simulink model "Neighborhood"  (R2024b)
settings: Solver=VariableStepAuto  StartTime=0.0  StopTime=20  RelTol=1e-3
undefined symbols (not defined in the file): A, A0_obv, adj, agent_1, agent_2, agent_3, agent_4, agent_5, agent_6, agent_noise_sensitivity_1, agent_noise_sensitivity_2, agent_noise_sensitivity_3, agent_noise_sensitivity_4, agent_noise_sensitivity_5, agent_noise_sensitivity_6, B, B0_obv, c, C, C0_obv, D, D0_obv, F, G, K, K0, noise_sensitivity, noise_ts
settings Model: Creator=Ivan  LastModifiedBy=Ivan

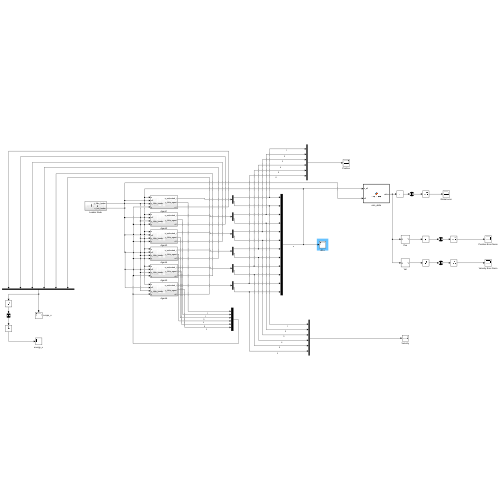
[thumbnail: Simulink's stored preview of the top-level diagram]
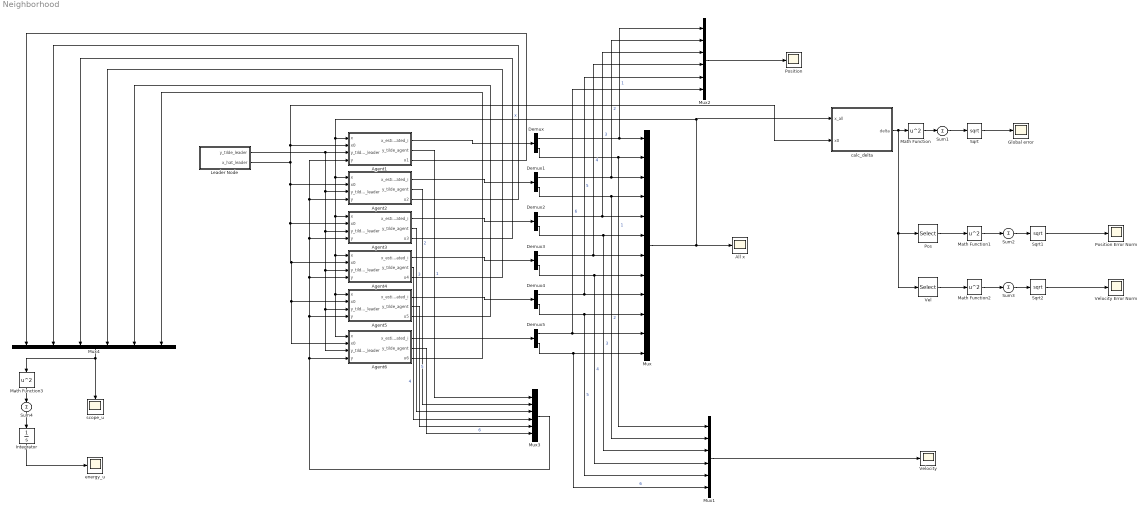
== system Neighborhood ==
  Agent1 : Subsystem
  Agent2 : Subsystem
  Agent3 : Subsystem
  Agent4 : Subsystem
  Agent5 : Subsystem
  Agent6 : Subsystem
  All x : Scope
  Demux{,1..5} (6 alike) : Demux  Outputs=2
  Global error : Scope
  Integrator : Integrator
  Leader Node : Subsystem
  Math Function{,1..3} (4 alike) : Math  Operator=square
  Mux : Mux  Inputs=12
  Mux{1..4} (4 alike) : Mux  Inputs=6
  Pos : Selector  NumberOfDimensions=2  InputPortWidth=3  IndexOptions=Index vector (dialog),Select all  Indices=[1],1  OutputSizes=1,1
  Position : Scope
  "Position Error Norm " : Scope
  Sqrt : Sqrt
  Sqrt1 : Sqrt
  Sqrt2 : Sqrt
  Sum{1..4} (4 alike) : Sum  Inputs=1
  Vel : Selector  NumberOfDimensions=2  InputPortWidth=3  IndexOptions=Index vector (dialog),Select all  Indices=[2],1  OutputSizes=1,1
  Velocity : Scope
  Velocity Error Norm : Scope
  calc_delta : MATLAB Function  TreatAsAtomicUnit=on
  energy_u : Scope
  scope_u : Scope
  wires:
  Demux1/2 -> Mux1/2, Mux/4  "2"
  Demux/1 -> Mux2/1, Mux/1  "1"
  Demux4/2 -> Mux1/5, Mux/10  "5"
  Demux/2 -> Mux/2, Mux1/1  "1"
  Demux1/1 -> Mux2/2, Mux/3  "2"
  Demux2/2 -> Mux1/3, Mux/6  "3"
  Demux4/1 -> Mux2/5, Mux/9  "5"
  Demux2/1 -> Mux/5, Mux2/3  "3"
  Demux3/2 -> Mux1/4, Mux/8  "4"
  Mux2/1 -> Position/1
  Mux1/1 -> Velocity/1
  Demux5/1 -> Mux2/6, Mux/11  "6"
  Demux5/2 -> Mux1/6, Mux/12  "6"
  Leader Node/2(x_hat_leader) -> calc_delta/2(x0), Agent1/2(x0), Agent2/2(x0), Agent3/2(x0), Agent4/2(x0), Agent6/2(x0), Agent5/2(x0)
  Mux/1 -> All x/1, calc_delta/1(x_all), Agent1/1(x), Agent2/1(x), Agent3/1(x), Agent4/1(x), Agent6/1(x), Agent5/1(x)  "x"
  Agent1/1(x_estimated_i) -> Demux/1
  Demux3/1 -> Mux2/4, Mux/7  "4"
  Agent2/1(x_estimated_i) -> Demux1/1
  Agent3/1(x_estimated_i) -> Demux2/1
  Agent4/1(x_estimated_i) -> Demux3/1
  Agent5/1(x_estimated_i) -> Demux4/1
  Agent6/1(x_estimated_i) -> Demux5/1
  Leader Node/1(y_tilde_leader) -> Agent2/3(y_tilde_leader), Agent3/3(y_tilde_leader), Agent4/3(y_tilde_leader), Agent6/3(y_tilde_leader), Agent5/3(y_tilde_leader), Agent1/3(y_tilde_leader)
  Agent1/2(y_tilde_agent) -> Mux3/1  "1"
  Agent2/2(y_tilde_agent) -> Mux3/2  "2"
  Agent3/2(y_tilde_agent) -> Mux3/3  "3"
  Agent4/2(y_tilde_agent) -> Mux3/4  "4"
  Agent5/2(y_tilde_agent) -> Mux3/5  "5"
  Agent6/2(y_tilde_agent) -> Mux3/6  "6"
  Mux3/1 -> Agent5/4(y), Agent4/4(y), Agent3/4(y), Agent2/4(y), Agent1/4(y), Agent6/4(y)
  Math Function2/1 -> Sum3/1
  Vel/1 -> Math Function2/1
  Sqrt/1 -> Global error/1
  Sum1/1 -> Sqrt/1
  Math Function1/1 -> Sum2/1
  Pos/1 -> Math Function1/1
  calc_delta/1(delta) -> Vel/1, Pos/1, Math Function/1
  Math Function/1 -> Sum1/1
  Sqrt2/1 -> Velocity Error Norm/1
  Sum3/1 -> Sqrt2/1
  Sum2/1 -> Sqrt1/1
  Sqrt1/1 -> "Position Error Norm "/1
  Sum4/1 -> Integrator/1
  Math Function3/1 -> Sum4/1
  Integrator/1 -> energy_u/1
  Mux4/1 -> scope_u/1, Math Function3/1
  Agent1/3(u1) -> Mux4/1
  Agent2/3(u2) -> Mux4/2
  Agent3/3(u3) -> Mux4/3
  Agent4/3(u4) -> Mux4/4
  Agent5/3(u5) -> Mux4/5
  Agent6/3(u6) -> Mux4/6

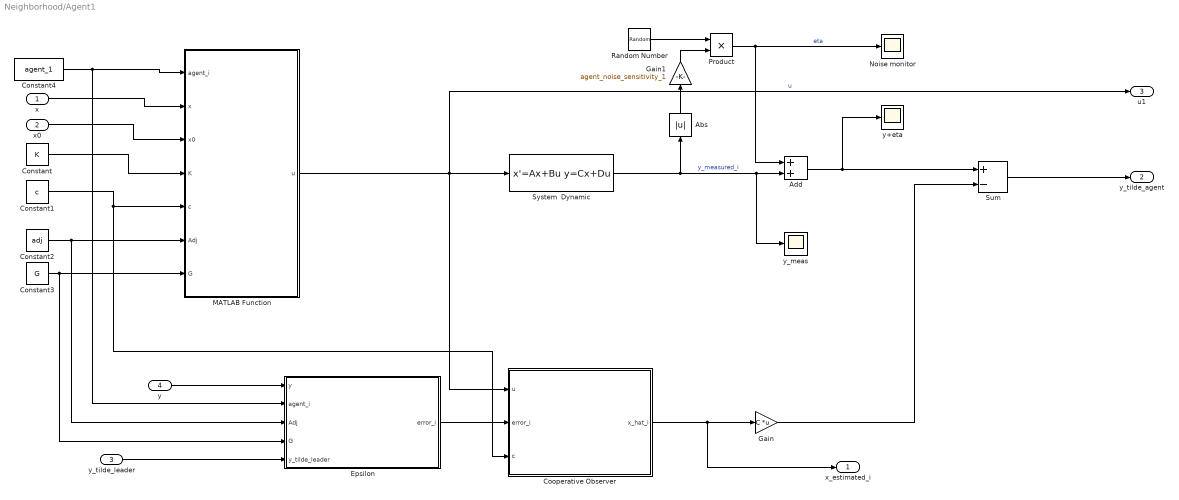
== system Neighborhood/Agent1 ==
  x : Inport
  x0 : Inport  Port=2
  y_tilde_leader : Inport  Port=3
  y : Inport  Port=4
  Abs : Abs  SaturateOnIntegerOverflow=off
  Add : Sum
  Constant : Constant  Value=K  VectorParams1D=off
  Constant1 : Constant  Value=c
  Constant2 : Constant  Value=adj
  Constant3 : Constant  Value=G
  Constant4 : Constant  Value=agent_1  VectorParams1D=off
  Cooperative Observer : Subsystem
  Epsilon : MATLAB Function  TreatAsAtomicUnit=on
  Gain : Gain  Gain=C  Multiplication=Matrix(K*u)
  Gain1 : Gain  Gain=agent_noise_sensitivity_1
  MATLAB Function : MATLAB Function  TreatAsAtomicUnit=on
  Noise monitor : Scope
  Product : Product
  Random Number : RandomNumber  SampleTime=noise_ts
  Sum : Sum  Inputs=+-
  System  Dynamic : StateSpace  A=(A-B*K0)  B=B  C=C  D=0  InitialCondition=0
  y+eta : Scope
  y_meas : Scope
  x_estimated_i : Outport
  y_tilde_agent : Outport  Port=2
  u1 : Outport  Port=3
  wires:
  x/1 -> MATLAB Function/2(x)
  Constant3/1 -> Epsilon/4(G), MATLAB Function/7(G)
  Constant1/1 -> Cooperative Observer/3(c), MATLAB Function/5(c)
  Constant/1 -> MATLAB Function/4(K)
  Constant4/1 -> Epsilon/2(agent_i), MATLAB Function/1(agent_i)
  Constant2/1 -> MATLAB Function/6(Adj), Epsilon/3(Adj)
  MATLAB Function/1(u) -> u1/1, Cooperative Observer/1(u), System  Dynamic/1  "u"
  x0/1 -> MATLAB Function/3(x0)
  y/1 -> Epsilon/1(y)
  y_tilde_leader/1 -> Epsilon/5(y_tilde_leader)
  Epsilon/1(error_i) -> Cooperative Observer/2(error_i)
  Cooperative Observer/1(x_hat_i) -> x_estimated_i/1, Gain/1
  System  Dynamic/1 -> Abs/1, y_meas/1, Add/2  "y_measured_i"
  Gain/1 -> Sum/2
  Sum/1 -> y_tilde_agent/1
  Product/1 -> Noise monitor/1, Add/1  "eta"
  Gain1/1 -> Product/2
  Abs/1 -> Gain1/1
  Random Number/1 -> Product/1
  Add/1 -> y+eta/1, Sum/1

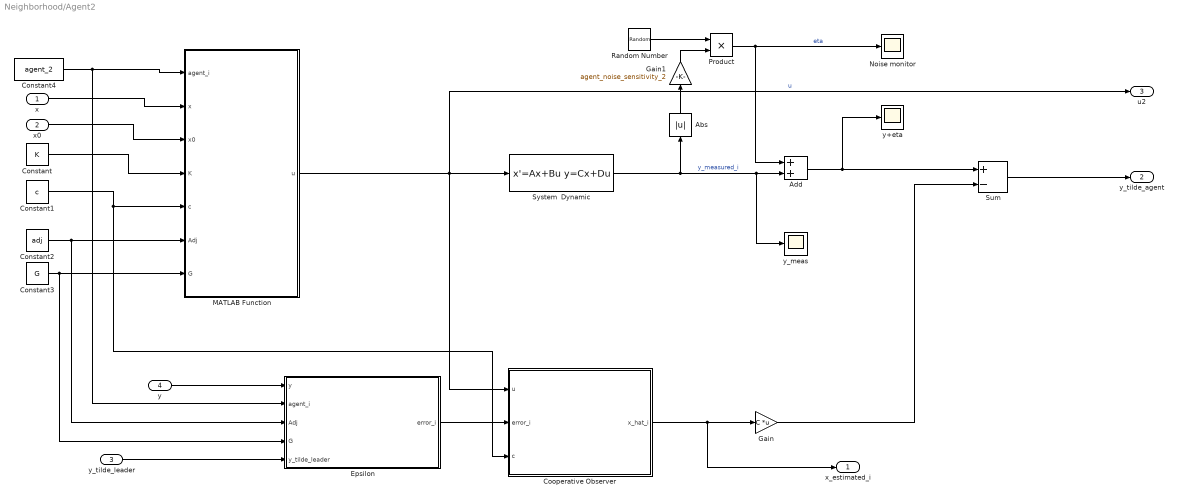
== system Neighborhood/Agent2 ==
  x : Inport
  x0 : Inport  Port=2
  y_tilde_leader : Inport  Port=3
  y : Inport  Port=4
  Abs : Abs  SaturateOnIntegerOverflow=off
  Add : Sum
  Constant : Constant  Value=K  VectorParams1D=off
  Constant1 : Constant  Value=c
  Constant2 : Constant  Value=adj
  Constant3 : Constant  Value=G
  Constant4 : Constant  Value=agent_2  VectorParams1D=off
  Cooperative Observer : Subsystem
  Epsilon : MATLAB Function  TreatAsAtomicUnit=on
  Gain : Gain  Gain=C  Multiplication=Matrix(K*u)
  Gain1 : Gain  Gain=agent_noise_sensitivity_2
  MATLAB Function : MATLAB Function  TreatAsAtomicUnit=on
  Noise monitor : Scope
  Product : Product
  Random Number : RandomNumber  SampleTime=noise_ts
  Sum : Sum  Inputs=+-
  System  Dynamic : StateSpace  A=(A-B*K0)  B=B  C=C  D=0  InitialCondition=0
  y+eta : Scope
  y_meas : Scope
  x_estimated_i : Outport
  y_tilde_agent : Outport  Port=2
  u2 : Outport  Port=3
  wires:
  x/1 -> MATLAB Function/2(x)
  Constant3/1 -> Epsilon/4(G), MATLAB Function/7(G)
  Constant1/1 -> Cooperative Observer/3(c), MATLAB Function/5(c)
  Constant/1 -> MATLAB Function/4(K)
  Constant4/1 -> Epsilon/2(agent_i), MATLAB Function/1(agent_i)
  Constant2/1 -> MATLAB Function/6(Adj), Epsilon/3(Adj)
  MATLAB Function/1(u) -> u2/1, Cooperative Observer/1(u), System  Dynamic/1  "u"
  x0/1 -> MATLAB Function/3(x0)
  y/1 -> Epsilon/1(y)
  y_tilde_leader/1 -> Epsilon/5(y_tilde_leader)
  Epsilon/1(error_i) -> Cooperative Observer/2(error_i)
  Cooperative Observer/1(x_hat_i) -> x_estimated_i/1, Gain/1
  System  Dynamic/1 -> Abs/1, y_meas/1, Add/2  "y_measured_i"
  Gain/1 -> Sum/2
  Sum/1 -> y_tilde_agent/1
  Product/1 -> Noise monitor/1, Add/1  "eta"
  Gain1/1 -> Product/2
  Abs/1 -> Gain1/1
  Random Number/1 -> Product/1
  Add/1 -> y+eta/1, Sum/1

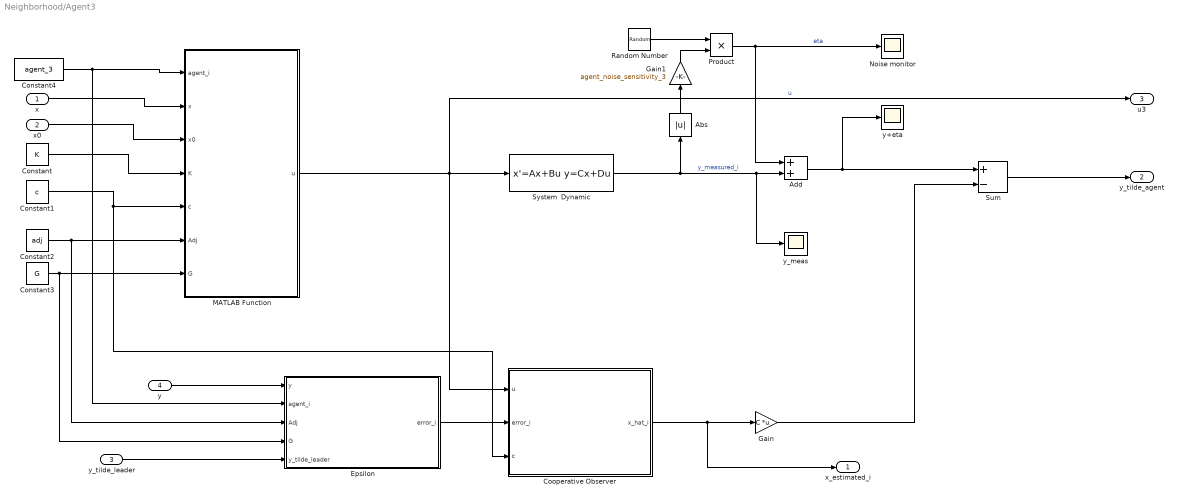
== system Neighborhood/Agent3 ==
  x : Inport
  x0 : Inport  Port=2
  y_tilde_leader : Inport  Port=3
  y : Inport  Port=4
  Abs : Abs  SaturateOnIntegerOverflow=off
  Add : Sum
  Constant : Constant  Value=K  VectorParams1D=off
  Constant1 : Constant  Value=c
  Constant2 : Constant  Value=adj
  Constant3 : Constant  Value=G
  Constant4 : Constant  Value=agent_3  VectorParams1D=off
  Cooperative Observer : Subsystem
  Epsilon : MATLAB Function  TreatAsAtomicUnit=on
  Gain : Gain  Gain=C  Multiplication=Matrix(K*u)
  Gain1 : Gain  Gain=agent_noise_sensitivity_3
  MATLAB Function : MATLAB Function  TreatAsAtomicUnit=on
  Noise monitor : Scope
  Product : Product
  Random Number : RandomNumber  SampleTime=noise_ts
  Sum : Sum  Inputs=+-
  System  Dynamic : StateSpace  A=(A-B*K0)  B=B  C=C  D=0  InitialCondition=0
  y+eta : Scope
  y_meas : Scope
  x_estimated_i : Outport
  y_tilde_agent : Outport  Port=2
  u3 : Outport  Port=3
  wires:
  x/1 -> MATLAB Function/2(x)
  Constant3/1 -> Epsilon/4(G), MATLAB Function/7(G)
  Constant1/1 -> Cooperative Observer/3(c), MATLAB Function/5(c)
  Constant/1 -> MATLAB Function/4(K)
  Constant4/1 -> Epsilon/2(agent_i), MATLAB Function/1(agent_i)
  Constant2/1 -> MATLAB Function/6(Adj), Epsilon/3(Adj)
  MATLAB Function/1(u) -> u3/1, Cooperative Observer/1(u), System  Dynamic/1  "u"
  x0/1 -> MATLAB Function/3(x0)
  y/1 -> Epsilon/1(y)
  y_tilde_leader/1 -> Epsilon/5(y_tilde_leader)
  Epsilon/1(error_i) -> Cooperative Observer/2(error_i)
  Cooperative Observer/1(x_hat_i) -> x_estimated_i/1, Gain/1
  System  Dynamic/1 -> Abs/1, y_meas/1, Add/2  "y_measured_i"
  Gain/1 -> Sum/2
  Sum/1 -> y_tilde_agent/1
  Product/1 -> Noise monitor/1, Add/1  "eta"
  Gain1/1 -> Product/2
  Abs/1 -> Gain1/1
  Random Number/1 -> Product/1
  Add/1 -> y+eta/1, Sum/1

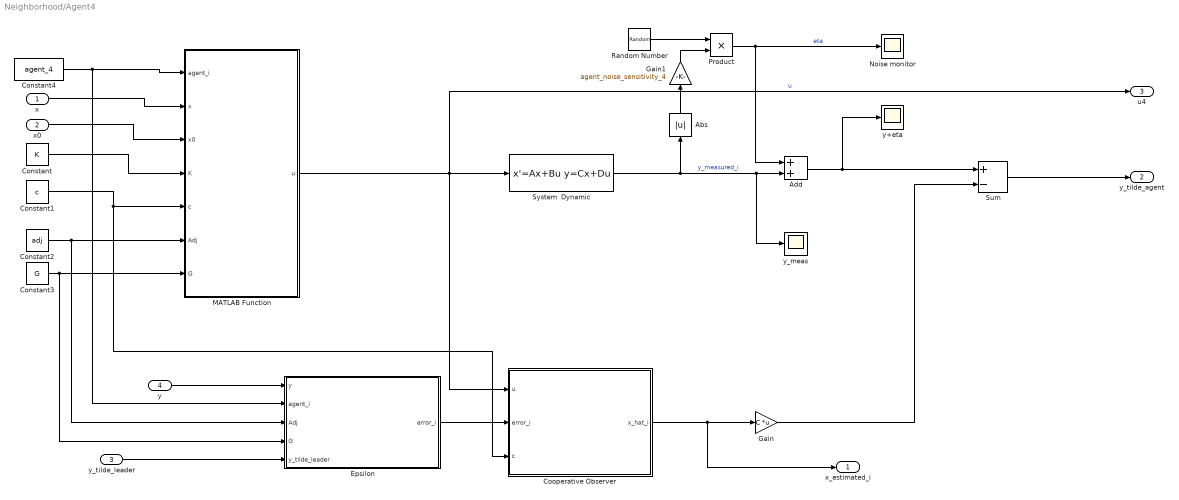
== system Neighborhood/Agent4 ==
  x : Inport
  x0 : Inport  Port=2
  y_tilde_leader : Inport  Port=3
  y : Inport  Port=4
  Abs : Abs  SaturateOnIntegerOverflow=off
  Add : Sum
  Constant : Constant  Value=K  VectorParams1D=off
  Constant1 : Constant  Value=c
  Constant2 : Constant  Value=adj
  Constant3 : Constant  Value=G
  Constant4 : Constant  Value=agent_4  VectorParams1D=off
  Cooperative Observer : Subsystem
  Epsilon : MATLAB Function  TreatAsAtomicUnit=on
  Gain : Gain  Gain=C  Multiplication=Matrix(K*u)
  Gain1 : Gain  Gain=agent_noise_sensitivity_4
  MATLAB Function : MATLAB Function  TreatAsAtomicUnit=on
  Noise monitor : Scope
  Product : Product
  Random Number : RandomNumber  SampleTime=noise_ts
  Sum : Sum  Inputs=+-
  System  Dynamic : StateSpace  A=(A-B*K0)  B=B  C=C  D=0  InitialCondition=0
  y+eta : Scope
  y_meas : Scope
  x_estimated_i : Outport
  y_tilde_agent : Outport  Port=2
  u4 : Outport  Port=3
  wires:
  x/1 -> MATLAB Function/2(x)
  Constant3/1 -> Epsilon/4(G), MATLAB Function/7(G)
  Constant1/1 -> Cooperative Observer/3(c), MATLAB Function/5(c)
  Constant/1 -> MATLAB Function/4(K)
  Constant4/1 -> Epsilon/2(agent_i), MATLAB Function/1(agent_i)
  Constant2/1 -> MATLAB Function/6(Adj), Epsilon/3(Adj)
  MATLAB Function/1(u) -> u4/1, Cooperative Observer/1(u), System  Dynamic/1  "u"
  x0/1 -> MATLAB Function/3(x0)
  y/1 -> Epsilon/1(y)
  y_tilde_leader/1 -> Epsilon/5(y_tilde_leader)
  Epsilon/1(error_i) -> Cooperative Observer/2(error_i)
  Cooperative Observer/1(x_hat_i) -> x_estimated_i/1, Gain/1
  System  Dynamic/1 -> Abs/1, y_meas/1, Add/2  "y_measured_i"
  Gain/1 -> Sum/2
  Sum/1 -> y_tilde_agent/1
  Product/1 -> Noise monitor/1, Add/1  "eta"
  Gain1/1 -> Product/2
  Abs/1 -> Gain1/1
  Random Number/1 -> Product/1
  Add/1 -> y+eta/1, Sum/1

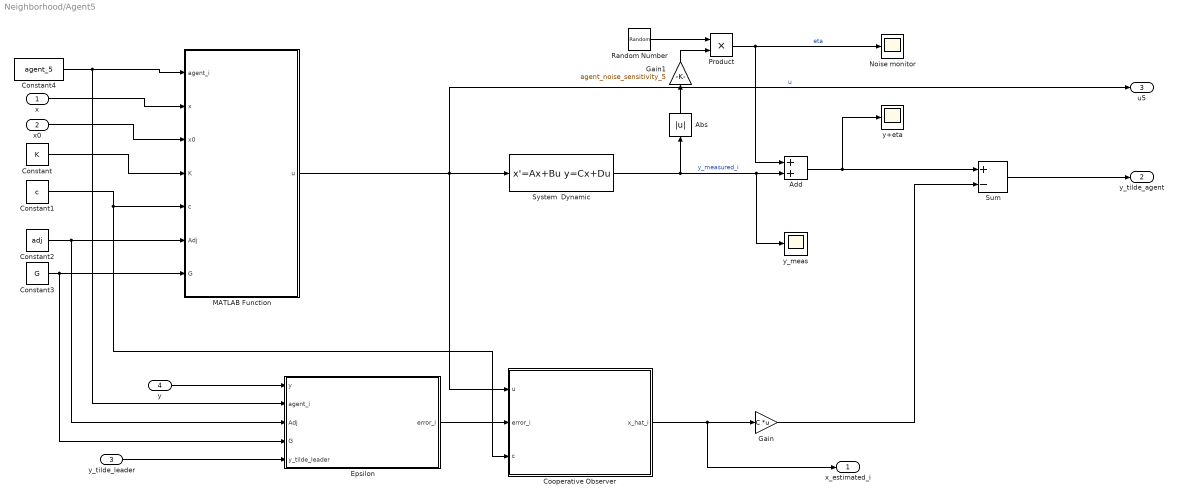
== system Neighborhood/Agent5 ==
  x : Inport
  x0 : Inport  Port=2
  y_tilde_leader : Inport  Port=3
  y : Inport  Port=4
  Abs : Abs  SaturateOnIntegerOverflow=off
  Add : Sum
  Constant : Constant  Value=K  VectorParams1D=off
  Constant1 : Constant  Value=c
  Constant2 : Constant  Value=adj
  Constant3 : Constant  Value=G
  Constant4 : Constant  Value=agent_5  VectorParams1D=off
  Cooperative Observer : Subsystem
  Epsilon : MATLAB Function  TreatAsAtomicUnit=on
  Gain : Gain  Gain=C  Multiplication=Matrix(K*u)
  Gain1 : Gain  Gain=agent_noise_sensitivity_5
  MATLAB Function : MATLAB Function  TreatAsAtomicUnit=on
  Noise monitor : Scope
  Product : Product
  Random Number : RandomNumber  SampleTime=noise_ts
  Sum : Sum  Inputs=+-
  System  Dynamic : StateSpace  A=(A-B*K0)  B=B  C=C  D=0  InitialCondition=0
  y+eta : Scope
  y_meas : Scope
  x_estimated_i : Outport
  y_tilde_agent : Outport  Port=2
  u5 : Outport  Port=3
  wires:
  x/1 -> MATLAB Function/2(x)
  Constant3/1 -> Epsilon/4(G), MATLAB Function/7(G)
  Constant1/1 -> Cooperative Observer/3(c), MATLAB Function/5(c)
  Constant/1 -> MATLAB Function/4(K)
  Constant4/1 -> Epsilon/2(agent_i), MATLAB Function/1(agent_i)
  Constant2/1 -> MATLAB Function/6(Adj), Epsilon/3(Adj)
  MATLAB Function/1(u) -> u5/1, Cooperative Observer/1(u), System  Dynamic/1  "u"
  x0/1 -> MATLAB Function/3(x0)
  y/1 -> Epsilon/1(y)
  y_tilde_leader/1 -> Epsilon/5(y_tilde_leader)
  Epsilon/1(error_i) -> Cooperative Observer/2(error_i)
  Cooperative Observer/1(x_hat_i) -> x_estimated_i/1, Gain/1
  System  Dynamic/1 -> Abs/1, y_meas/1, Add/2  "y_measured_i"
  Gain/1 -> Sum/2
  Sum/1 -> y_tilde_agent/1
  Product/1 -> Noise monitor/1, Add/1  "eta"
  Gain1/1 -> Product/2
  Abs/1 -> Gain1/1
  Random Number/1 -> Product/1
  Add/1 -> y+eta/1, Sum/1

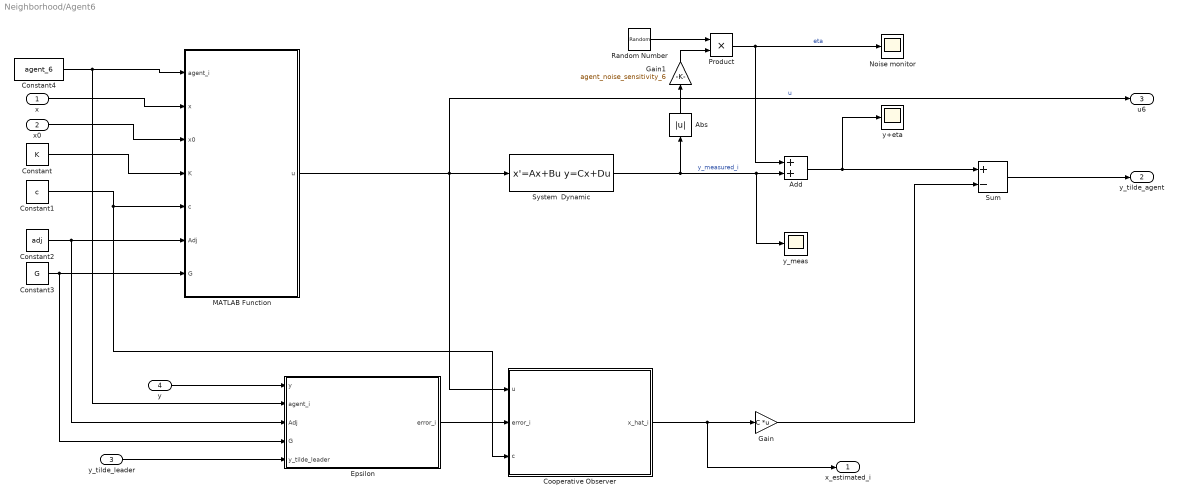
== system Neighborhood/Agent6 ==
  x : Inport
  x0 : Inport  Port=2
  y_tilde_leader : Inport  Port=3
  y : Inport  Port=4
  Abs : Abs  SaturateOnIntegerOverflow=off
  Add : Sum
  Constant : Constant  Value=K  VectorParams1D=off
  Constant1 : Constant  Value=c
  Constant2 : Constant  Value=adj
  Constant3 : Constant  Value=G
  Constant4 : Constant  Value=agent_6  VectorParams1D=off
  Cooperative Observer : Subsystem
  Epsilon : MATLAB Function  TreatAsAtomicUnit=on
  Gain : Gain  Gain=C  Multiplication=Matrix(K*u)
  Gain1 : Gain  Gain=agent_noise_sensitivity_6
  MATLAB Function : MATLAB Function  TreatAsAtomicUnit=on
  Noise monitor : Scope
  Product : Product
  Random Number : RandomNumber  SampleTime=noise_ts
  Sum : Sum  Inputs=+-
  System  Dynamic : StateSpace  A=(A-B*K0)  B=B  C=C  D=0  InitialCondition=0
  y+eta : Scope
  y_meas : Scope
  x_estimated_i : Outport
  y_tilde_agent : Outport  Port=2
  u6 : Outport  Port=3
  wires:
  x/1 -> MATLAB Function/2(x)
  Constant3/1 -> Epsilon/4(G), MATLAB Function/7(G)
  Constant1/1 -> Cooperative Observer/3(c), MATLAB Function/5(c)
  Constant/1 -> MATLAB Function/4(K)
  Constant4/1 -> Epsilon/2(agent_i), MATLAB Function/1(agent_i)
  Constant2/1 -> MATLAB Function/6(Adj), Epsilon/3(Adj)
  MATLAB Function/1(u) -> u6/1, Cooperative Observer/1(u), System  Dynamic/1  "u"
  x0/1 -> MATLAB Function/3(x0)
  y/1 -> Epsilon/1(y)
  y_tilde_leader/1 -> Epsilon/5(y_tilde_leader)
  Epsilon/1(error_i) -> Cooperative Observer/2(error_i)
  Cooperative Observer/1(x_hat_i) -> x_estimated_i/1, Gain/1
  System  Dynamic/1 -> Abs/1, y_meas/1, Add/2  "y_measured_i"
  Gain/1 -> Sum/2
  Sum/1 -> y_tilde_agent/1
  Product/1 -> Noise monitor/1, Add/1  "eta"
  Gain1/1 -> Product/2
  Abs/1 -> Gain1/1
  Random Number/1 -> Product/1
  Add/1 -> y+eta/1, Sum/1

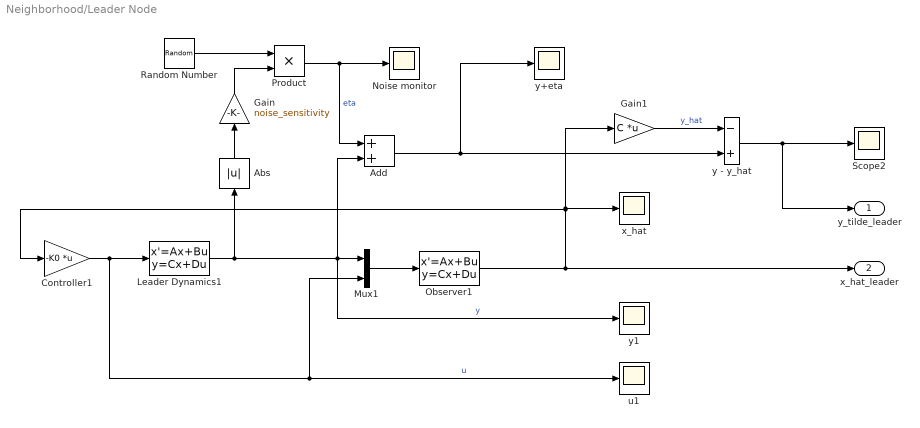
== system Neighborhood/Leader Node ==
  Abs : Abs  SaturateOnIntegerOverflow=off
  Add : Sum
  Controller1 : Gain  Gain=-K0  Multiplication=Matrix(K*u)
  Gain : Gain  Gain=noise_sensitivity
  Gain1 : Gain  Gain=C  Multiplication=Matrix(K*u)
  Leader Dynamics1 : StateSpace  A=A  B=B  C=C  D=D  InitialCondition=[0 100]'
  Mux1 : Mux  Inputs=2
  Noise monitor : Scope
  Observer1 : StateSpace  A=A0_obv  B=B0_obv  C=C0_obv  D=D0_obv  InitialCondition=0
  Product : Product
  Random Number : RandomNumber  SampleTime=noise_ts
  Scope2 : Scope
  u1 : Scope
  x_hat : Scope
  y - y_hat : Sum  Inputs=-+
  y+eta : Scope
  y1 : Scope
  y_tilde_leader : Outport
  x_hat_leader : Outport  Port=2
  wires:
  y - y_hat/1 -> y_tilde_leader/1, Scope2/1
  Controller1/1 -> Mux1/2, u1/1, Leader Dynamics1/1  "u"
  Observer1/1 -> x_hat_leader/1, x_hat/1, Gain1/1, Controller1/1
  Mux1/1 -> Observer1/1
  Gain1/1 -> y - y_hat/1  "y_hat"
  Leader Dynamics1/1 -> Add/2, y1/1, Mux1/1, Abs/1  "y"
  Add/1 -> y - y_hat/2, y+eta/1
  Abs/1 -> Gain/1
  Random Number/1 -> Product/1
  Gain/1 -> Product/2
  Product/1 -> Noise monitor/1, Add/1  "eta"

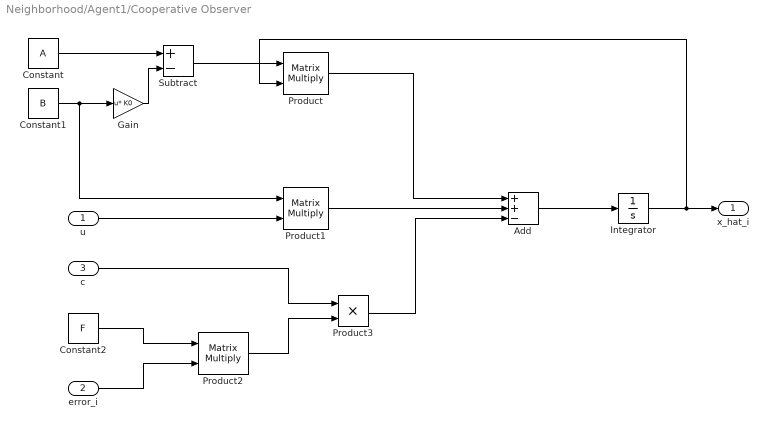
== system Neighborhood/Agent1/Cooperative Observer ==
  u : Inport
  error_i : Inport  Port=2
  c : Inport  Port=3
  Add : Sum  Inputs=++-
  Constant : Constant  Value=A
  Constant1 : Constant  Value=B
  Constant2 : Constant  Value=F
  Gain : Gain  Gain=K0  Multiplication=Matrix(u*K)
  Integrator : Integrator
  Product : Product  Multiplication=Matrix(*)
  Product1 : Product  Multiplication=Matrix(*)
  Product2 : Product  Multiplication=Matrix(*)
  Product3 : Product
  Subtract : Sum  Inputs=+-
  x_hat_i : Outport
  wires:
  Constant1/1 -> Product1/1, Gain/1
  Gain/1 -> Subtract/2
  Constant/1 -> Subtract/1
  u/1 -> Product1/2
  Subtract/1 -> Product/1
  Product/1 -> Add/1
  Product1/1 -> Add/2
  Add/1 -> Integrator/1
  Integrator/1 -> Product/2, x_hat_i/1
  error_i/1 -> Product2/2
  Constant2/1 -> Product2/1
  c/1 -> Product3/1
  Product2/1 -> Product3/2
  Product3/1 -> Add/3

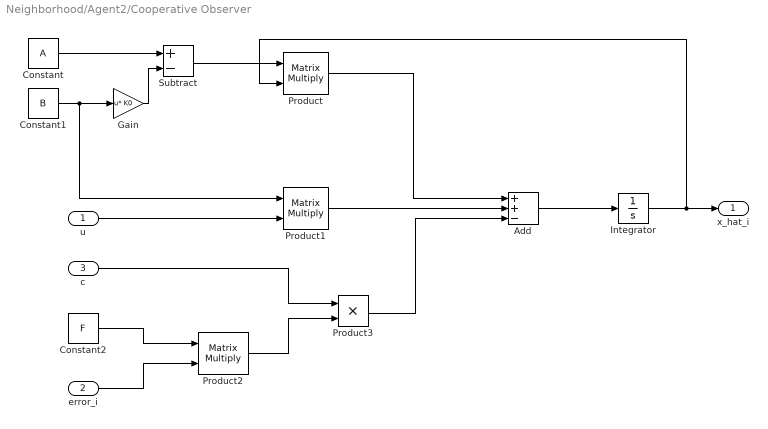
== system Neighborhood/Agent2/Cooperative Observer ==
  u : Inport
  error_i : Inport  Port=2
  c : Inport  Port=3
  Add : Sum  Inputs=++-
  Constant : Constant  Value=A
  Constant1 : Constant  Value=B
  Constant2 : Constant  Value=F
  Gain : Gain  Gain=K0  Multiplication=Matrix(u*K)
  Integrator : Integrator
  Product : Product  Multiplication=Matrix(*)
  Product1 : Product  Multiplication=Matrix(*)
  Product2 : Product  Multiplication=Matrix(*)
  Product3 : Product
  Subtract : Sum  Inputs=+-
  x_hat_i : Outport
  wires:
  Constant1/1 -> Product1/1, Gain/1
  Gain/1 -> Subtract/2
  Constant/1 -> Subtract/1
  u/1 -> Product1/2
  Subtract/1 -> Product/1
  Product/1 -> Add/1
  Product1/1 -> Add/2
  Add/1 -> Integrator/1
  Integrator/1 -> Product/2, x_hat_i/1
  error_i/1 -> Product2/2
  Constant2/1 -> Product2/1
  c/1 -> Product3/1
  Product2/1 -> Product3/2
  Product3/1 -> Add/3

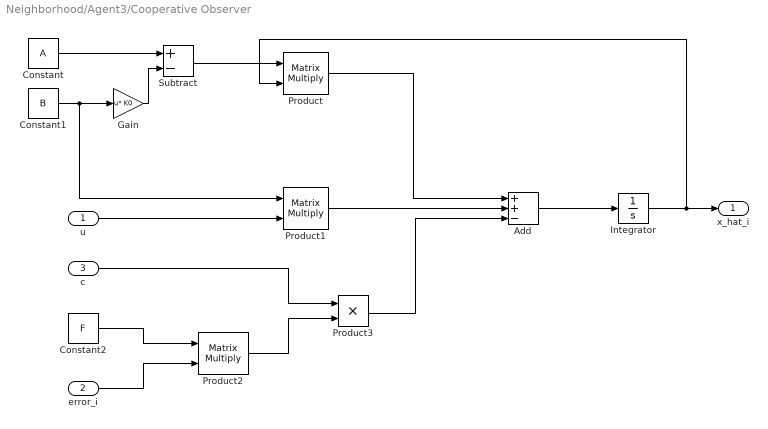
== system Neighborhood/Agent3/Cooperative Observer ==
  u : Inport
  error_i : Inport  Port=2
  c : Inport  Port=3
  Add : Sum  Inputs=++-
  Constant : Constant  Value=A
  Constant1 : Constant  Value=B
  Constant2 : Constant  Value=F
  Gain : Gain  Gain=K0  Multiplication=Matrix(u*K)
  Integrator : Integrator
  Product : Product  Multiplication=Matrix(*)
  Product1 : Product  Multiplication=Matrix(*)
  Product2 : Product  Multiplication=Matrix(*)
  Product3 : Product
  Subtract : Sum  Inputs=+-
  x_hat_i : Outport
  wires:
  Constant1/1 -> Product1/1, Gain/1
  Gain/1 -> Subtract/2
  Constant/1 -> Subtract/1
  u/1 -> Product1/2
  Subtract/1 -> Product/1
  Product/1 -> Add/1
  Product1/1 -> Add/2
  Add/1 -> Integrator/1
  Integrator/1 -> Product/2, x_hat_i/1
  error_i/1 -> Product2/2
  Constant2/1 -> Product2/1
  c/1 -> Product3/1
  Product2/1 -> Product3/2
  Product3/1 -> Add/3

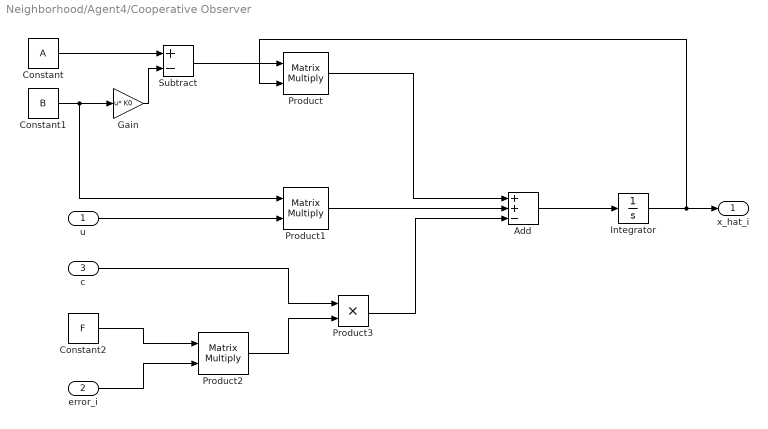
== system Neighborhood/Agent4/Cooperative Observer ==
  u : Inport
  error_i : Inport  Port=2
  c : Inport  Port=3
  Add : Sum  Inputs=++-
  Constant : Constant  Value=A
  Constant1 : Constant  Value=B
  Constant2 : Constant  Value=F
  Gain : Gain  Gain=K0  Multiplication=Matrix(u*K)
  Integrator : Integrator
  Product : Product  Multiplication=Matrix(*)
  Product1 : Product  Multiplication=Matrix(*)
  Product2 : Product  Multiplication=Matrix(*)
  Product3 : Product
  Subtract : Sum  Inputs=+-
  x_hat_i : Outport
  wires:
  Constant1/1 -> Product1/1, Gain/1
  Gain/1 -> Subtract/2
  Constant/1 -> Subtract/1
  u/1 -> Product1/2
  Subtract/1 -> Product/1
  Product/1 -> Add/1
  Product1/1 -> Add/2
  Add/1 -> Integrator/1
  Integrator/1 -> Product/2, x_hat_i/1
  error_i/1 -> Product2/2
  Constant2/1 -> Product2/1
  c/1 -> Product3/1
  Product2/1 -> Product3/2
  Product3/1 -> Add/3

== system Neighborhood/Agent5/Cooperative Observer ==
  u : Inport
  error_i : Inport  Port=2
  c : Inport  Port=3
  Add : Sum  Inputs=++-
  Constant : Constant  Value=A
  Constant1 : Constant  Value=B
  Constant2 : Constant  Value=F
  Gain : Gain  Gain=K0  Multiplication=Matrix(u*K)
  Integrator : Integrator
  Product : Product  Multiplication=Matrix(*)
  Product1 : Product  Multiplication=Matrix(*)
  Product2 : Product  Multiplication=Matrix(*)
  Product3 : Product
  Subtract : Sum  Inputs=+-
  x_hat_i : Outport
  wires:
  Constant1/1 -> Product1/1, Gain/1
  Gain/1 -> Subtract/2
  Constant/1 -> Subtract/1
  u/1 -> Product1/2
  Subtract/1 -> Product/1
  Product/1 -> Add/1
  Product1/1 -> Add/2
  Add/1 -> Integrator/1
  Integrator/1 -> Product/2, x_hat_i/1
  error_i/1 -> Product2/2
  Constant2/1 -> Product2/1
  c/1 -> Product3/1
  Product2/1 -> Product3/2
  Product3/1 -> Add/3

== system Neighborhood/Agent6/Cooperative Observer ==
  u : Inport
  error_i : Inport  Port=2
  c : Inport  Port=3
  Add : Sum  Inputs=++-
  Constant : Constant  Value=A
  Constant1 : Constant  Value=B
  Constant2 : Constant  Value=F
  Gain : Gain  Gain=K0  Multiplication=Matrix(u*K)
  Integrator : Integrator
  Product : Product  Multiplication=Matrix(*)
  Product1 : Product  Multiplication=Matrix(*)
  Product2 : Product  Multiplication=Matrix(*)
  Product3 : Product
  Subtract : Sum  Inputs=+-
  x_hat_i : Outport
  wires:
  Constant1/1 -> Product1/1, Gain/1
  Gain/1 -> Subtract/2
  Constant/1 -> Subtract/1
  u/1 -> Product1/2
  Subtract/1 -> Product/1
  Product/1 -> Add/1
  Product1/1 -> Add/2
  Add/1 -> Integrator/1
  Integrator/1 -> Product/2, x_hat_i/1
  error_i/1 -> Product2/2
  Constant2/1 -> Product2/1
  c/1 -> Product3/1
  Product2/1 -> Product3/2
  Product3/1 -> Add/3

== matlab function Neighborhood/Agent5/Epsilon ==
  data: y input; error_i output; agent_i input; Adj input; G input; y_tilde_leader input
function error_i = fcn(y, agent_i, Adj, G, y_tilde_leader)

error = 0;
for j = 1:6
    error = error + Adj(agent_i,j)*(y(j)-y(agent_i)) + G(agent_i)*(y_tilde_leader - y(agent_i));
end
error_i = error;

== matlab function Neighborhood/Agent5/MATLAB Function ==
  data: agent_i input; u output; x input; x0 input; K input; c input; Adj input; G input
function u = controller_agent(agent_i, x, x0, K, c, Adj, G)

% N = number of agents
N = length(Adj);  

% Number of entries of x
order = 2;

% Get the i-th 2x1 vector from the 12x1 size array (12 = N * 2, without leader)
get_x = @(idx) x(idx*order - (order-1) : idx*order);

% Error towards leader (reference)
a = G(agent_i)*(x0 - get_x(agent_i));

% Consensus error among agents
epsilon_i = zeros(order, 1);
for j = 1:N
    epsilon_i = epsilon_i + Adj(agent_i, j) * (get_x(j) - get_x(agent_i));
end

% Total error
epsilon_i = epsilon_i + a;

% Control law
u = c*K*epsilon_i;

== matlab function Neighborhood/Agent6/Epsilon ==
  data: y input; error_i output; agent_i input; Adj input; G input; y_tilde_leader input
function error_i = fcn(y, agent_i, Adj, G, y_tilde_leader)

error = 0;
for j = 1:6
    error = error + Adj(agent_i,j)*(y(j)-y(agent_i)) + G(agent_i)*(y_tilde_leader - y(agent_i));
end
error_i = error;

== matlab function Neighborhood/Agent1/Epsilon ==
  data: y input; error_i output; agent_i input; Adj input; G input; y_tilde_leader input
function error_i = fcn(y, agent_i, Adj, G, y_tilde_leader)

error = 0;
for j = 1:6
    error = error + Adj(agent_i,j)*(y(j)-y(agent_i)) + G(agent_i)*(y_tilde_leader - y(agent_i));
end
error_i = error;

== matlab function Neighborhood/Agent6/MATLAB Function ==
  data: agent_i input; u output; x input; x0 input; K input; c input; Adj input; G input
function u = controller_agent(agent_i, x, x0, K, c, Adj, G)

% N = number of agents
N = length(Adj);  

% Number of entries of x
order = 2;

% Get the i-th 2x1 vector from the 12x1 size array (12 = N * 2, without leader)
get_x = @(idx) x(idx*order - (order-1) : idx*order);

% Error towards leader (reference)
a = G(agent_i)*(x0 - get_x(agent_i));

% Consensus error among agents
epsilon_i = zeros(order, 1);
for j = 1:N
    epsilon_i = epsilon_i + Adj(agent_i, j) * (get_x(j) - get_x(agent_i));
end

% Total error
epsilon_i = epsilon_i + a;

% Control law
u = c*K*epsilon_i;

== matlab function Neighborhood/calc_delta ==
  data: x_all input; delta output; x0 input
function delta = calc_delta(x_all, x0)
% x_all: vettore [12x1] (2 stati per ciascuno dei 6 follower)
% x0: vettore [2x1] (leader)

N = length(x_all)/2; % numero di follower
delta = zeros(2, N); % matrice [2x6]

for i = 1:N
    xi = x_all(2*i-1:2*i); % prendi x_i
    delta(:, i) = xi - x0; % errore rispetto al leader
end

%Uscita del blocco delta:
%È una matrice 2×6 (righe = [posizione; velocità], colonne = agenti)

== matlab function Neighborhood/Agent1/MATLAB Function ==
  data: agent_i input; u output; x input; x0 input; K input; c input; Adj input; G input
function u = controller_agent(agent_i, x, x0, K, c, Adj, G)

% N = number of agents
N = length(Adj);  

% Number of entries of x
order = 2;

% Get the i-th 2x1 vector from the 12x1 size array (12 = N * 2, without leader)
get_x = @(idx) x(idx*order - (order-1) : idx*order);

% Error towards leader (reference)
a = G(agent_i)*(x0 - get_x(agent_i));

% Consensus error among agents
epsilon_i = zeros(order, 1);
for j = 1:N
    epsilon_i = epsilon_i + Adj(agent_i, j) * (get_x(j) - get_x(agent_i));
end

% Total error
epsilon_i = epsilon_i + a;

% Control law
u = c*K*epsilon_i;

== matlab function Neighborhood/Agent2/Epsilon ==
  data: y input; error_i output; agent_i input; Adj input; G input; y_tilde_leader input
function error_i = fcn(y, agent_i, Adj, G, y_tilde_leader)

error = 0;
for j = 1:6
    error = error + Adj(agent_i,j)*(y(j)-y(agent_i)) + G(agent_i)*(y_tilde_leader - y(agent_i));
end
error_i = error;

== matlab function Neighborhood/Agent2/MATLAB Function ==
  data: agent_i input; u output; x input; x0 input; K input; c input; Adj input; G input
function u = controller_agent(agent_i, x, x0, K, c, Adj, G)

% N = number of agents
N = length(Adj);  

% Number of entries of x
order = 2;

% Get the i-th 2x1 vector from the 12x1 size array (12 = N * 2, without leader)
get_x = @(idx) x(idx*order - (order-1) : idx*order);

% Error towards leader (reference)
a = G(agent_i)*(x0 - get_x(agent_i));

% Consensus error among agents
epsilon_i = zeros(order, 1);
for j = 1:N
    epsilon_i = epsilon_i + Adj(agent_i, j) * (get_x(j) - get_x(agent_i));
end

% Total error
epsilon_i = epsilon_i + a;

% Control law
u = c*K*epsilon_i;

== matlab function Neighborhood/Agent3/Epsilon ==
  data: y input; error_i output; agent_i input; Adj input; G input; y_tilde_leader input
function error_i = fcn(y, agent_i, Adj, G, y_tilde_leader)

error = 0;
for j = 1:6
    error = error + Adj(agent_i,j)*(y(j)-y(agent_i)) + G(agent_i)*(y_tilde_leader - y(agent_i));
end
error_i = error;

== matlab function Neighborhood/Agent3/MATLAB Function ==
  data: agent_i input; u output; x input; x0 input; K input; c input; Adj input; G input
function u = controller_agent(agent_i, x, x0, K, c, Adj, G)

% N = number of agents
N = length(Adj);  

% Number of entries of x
order = 2;

% Get the i-th 2x1 vector from the 12x1 size array (12 = N * 2, without leader)
get_x = @(idx) x(idx*order - (order-1) : idx*order);

% Error towards leader (reference)
a = G(agent_i)*(x0 - get_x(agent_i));

% Consensus error among agents
epsilon_i = zeros(order, 1);
for j = 1:N
    epsilon_i = epsilon_i + Adj(agent_i, j) * (get_x(j) - get_x(agent_i));
end

% Total error
epsilon_i = epsilon_i + a;

% Control law
u = c*K*epsilon_i;

== matlab function Neighborhood/Agent4/Epsilon ==
  data: y input; error_i output; agent_i input; Adj input; G input; y_tilde_leader input
function error_i = fcn(y, agent_i, Adj, G, y_tilde_leader)

error = 0;
for j = 1:6
    error = error + Adj(agent_i,j)*(y(j)-y(agent_i)) + G(agent_i)*(y_tilde_leader - y(agent_i));
end
error_i = error;

== matlab function Neighborhood/Agent4/MATLAB Function ==
  data: agent_i input; u output; x input; x0 input; K input; c input; Adj input; G input
function u = controller_agent(agent_i, x, x0, K, c, Adj, G)

% N = number of agents
N = length(Adj);  

% Number of entries of x
order = 2;

% Get the i-th 2x1 vector from the 12x1 size array (12 = N * 2, without leader)
get_x = @(idx) x(idx*order - (order-1) : idx*order);

% Error towards leader (reference)
a = G(agent_i)*(x0 - get_x(agent_i));

% Consensus error among agents
epsilon_i = zeros(order, 1);
for j = 1:N
    epsilon_i = epsilon_i + Adj(agent_i, j) * (get_x(j) - get_x(agent_i));
end

% Total error
epsilon_i = epsilon_i + a;

% Control law
u = c*K*epsilon_i;
